simulink library "SADLib"  (R2023b)
settings: Solver=VariableStepAuto  StartTime=0.0  StopTime=10.0  RelTol=1e-3
values from neighbouring files (symbols this model uses):
  I = diag(Iv)    [InitDoubleSpin.m]    (also in InitLab03.m)
  invI = inv(I)    [InitDoubleSpin.m]    (also in InitLab03.m)
  w0 = [1e-6; 0.005; 0.2]    [InitDoubleSpin.m]    (also in InitLab03.m = [2*pi; 0.5; 1])
libraries: matrix_library x1
settings Model: Creator=elisa  LastModifiedBy=elisa

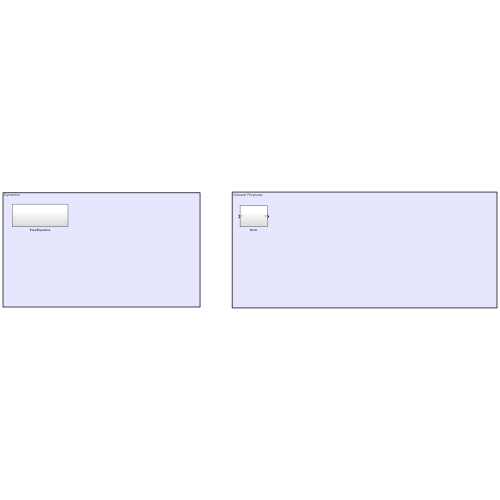
[thumbnail: Simulink's stored preview of the top-level diagram]
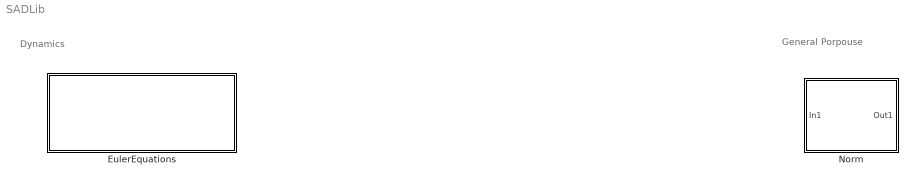
== system SADLib ==
  note: General Porpouse
  note: Dynamics
  EulerEquations : Subsystem
  Norm : Subsystem

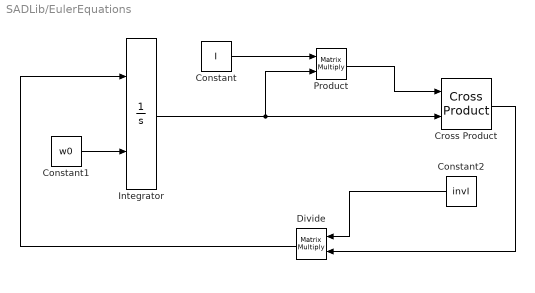
== system SADLib/EulerEquations ==
  Constant : Constant  Value=I
  Constant1 : Constant  Value=w0  VectorParams1D=off
  Constant2 : Constant  Value=invI
  Cross Product : matrix_library/Cross Product
  Divide : Product  Inputs=**  Multiplication=Matrix(*)
  Integrator : Integrator  InitialConditionSource=external
  Product : Product  Multiplication=Matrix(*)
  wires:
  Constant/1 -> Product/1
  Constant2/1 -> Divide/1
  Constant1/1 -> Integrator/2
  Integrator/1 -> Product/2, Cross Product/2
  Divide/1 -> Integrator/1
  Cross Product/1 -> Divide/2
  Product/1 -> Cross Product/1

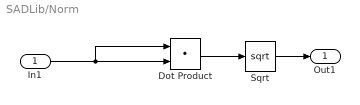
== system SADLib/Norm ==
  In1 : Inport
  Dot Product : DotProduct  OutDataTypeStr=Inherit: Inherit via internal rule
  Sqrt : Sqrt
  Out1 : Outport
  wires:
  Dot Product/1 -> Sqrt/1
  In1/1 -> Dot Product/1, Dot Product/2
  Sqrt/1 -> Out1/1
